simulink model "LCKIE"  (R2020b)
settings: Solver=FixedStepDiscrete  StartTime=0.0  StopTime=Inf  RelTol=1e-3
PostLoadFcn:
  | if any(exist('dsrtsu_mdlpostloadfcn', 'file') ~= 0), dsrtsu_mdlpostloadfcn('Execute', bdroot); end
InitFcn:
  | , if any(exist('rtifpga_mdlclblib', 'file') ~= 0), rtifpga_mdlclblib('Init', bdroot); end,
  | , if any(exist('dsmpb_private', 'file') ~= 0), dsmpb_private('dsmpb_mdlclblib', 'Init', bdroot); end,
PreSaveFcn:
  | , if any(exist('dsmpb_private', 'file') ~= 0), dsmpb_private('dsmpb_mdlclblib', 'PreSave', bdroot); end,
CloseFcn:
  | , if any(exist('dsmpb_private', 'file') ~= 0), dsmpb_private('dsmpb_mdlclblib', 'Close', bdroot); end,
settings Model: DataDictionary=HWA_DDs.sldd  RTICANMMDATA=struct('GeneralSetupData',struct('modelroot','E:\System\ADAS_BaseModel\ADAS_Store\Adas\VSM\LSSState\IE','generalsettings',struct('filesettings',struct('destfolder',struct('Name','RTICANMM_FILES','Check',1),'buildfolder',struct('Name','.','Check',1),'AbsDestfolder',struct('Name','E:\System\ADAS_BaseModel\ADAS_Store\Adas\VSM\LSSState\IE\RTICANMM_FILES'),'AbsBuildfolder',struct('Name','E:\System\ADAS_BaseModel\ADAS_Store\Adas\VSM\LSSState\IE'))),'options',struct('addpaths',1,'rmpaths',1,'addtrcexclusion',false,'cannavigator',struct('checkmonitoring',0),'show_usrtrc',0,'use_usrtrc',0),'advanced',struct('options',ones(1,100)),'MPSetup',{{}},'RTI',struct('Type','DSRT','Ver','4.4','Date','02-Nov-2020'),'modelname','LCKIE','block','LCKIE'))  DSRTSU_INTERNAL_RTIFPGA=170  Creator=GW00164938  LastModifiedBy=GW00164938
settings OptimizationCC: BlockReduction=off  ConditionallyExecuteInputs=off  OptimizeBlockIOStorage=off  BufferReuse=off
settings DebuggingCC: TasksWithSamePriorityMsg=none
settings HardwareCC: ProdBitPerPointer=32  ProdBitPerSizeT=32  ProdBitPerPtrDiffT=32  ProdLargestAtomicInteger=Integer  ProdWordSize=32  ProdHWDeviceType=Custom Processor->Custom
settings ModelReferenceCC: ModelReferenceNumInstancesAllowed=Single
settings SFSimCC: MATLABDynamicMemAlloc=off
settings RTWCC: Description=dSPACE Run-Time Target (for VEOS on Windows and ConfigurationDesk)  SystemTargetFile=dsrt.tlc  GenCodeOnly=on  MakeCommand=make_dsrt  TemplateMakefile=dsrt_default_tmf  RTWVerbose=off
settings CodeAppCC: MaxIdLength=128
settings STFCustomTargetCC: TargetLangStandard=C99 (ISO)  ParMdlRefBuildCompliant=on  ConcurrentExecutionCompliant=off  CPPClassGenCompliant=off  GRTInterface=off  SystemTargetFile=dsrt.tlc
settings GRTTargetCC: CompOptLevelCompliant=off  ConcurrentExecutionCompliant=off  CombineOutputUpdateFcns=off  MatFileLogging=off  CPPClassGenCompliant=off  UseToolchainInfoCompliant=off

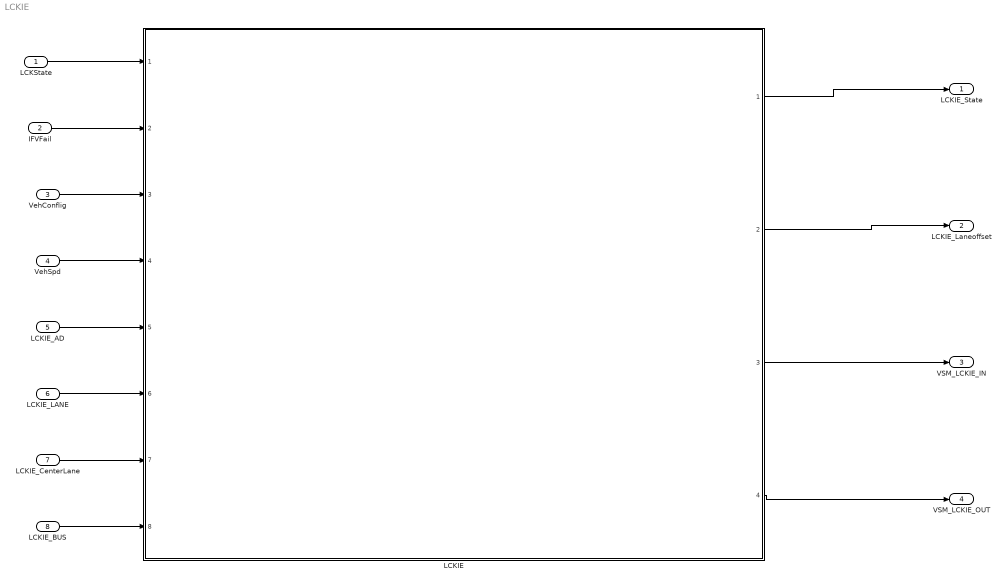
== system LCKIE ==
  LCKState : Inport
  IFVFail : Inport  Port=2
  VehConflig : Inport  Port=3
  VehSpd : Inport  Port=4
  LCKIE_AD : Inport  Port=5  OutDataTypeStr=Bus: LCKIE_AD  BusOutputAsStruct=on
  LCKIE_LANE : Inport  Port=6  OutDataTypeStr=Bus: LCKIE_Lane  BusOutputAsStruct=on
  LCKIE_CenterLane : Inport  Port=7  OutDataTypeStr=Bus: CenterLane  BusOutputAsStruct=on
  LCKIE_BUS : Inport  Port=8  OutDataTypeStr=Bus: TOS_LCKIE_BUS  BusOutputAsStruct=on
  LCKIE : Subsystem  ReferencedSubsystem=PvtSubSys_VSM_LCKIE
  LCKIE_State : Outport
  LCKIE_Laneoffset : Outport  Port=2
  VSM_LCKIE_IN : Outport  Port=3
  VSM_LCKIE_OUT : Outport  Port=4
  wires:
  LCKIE/1 -> LCKIE_State/1
  LCKIE/2 -> LCKIE_Laneoffset/1
  LCKIE/3 -> VSM_LCKIE_IN/1
  LCKIE/4 -> VSM_LCKIE_OUT/1
  VehConflig/1 -> LCKIE/3
  VehSpd/1 -> LCKIE/4
  LCKIE_AD/1 -> LCKIE/5
  LCKIE_CenterLane/1 -> LCKIE/7
  LCKIE_BUS/1 -> LCKIE/8
  IFVFail/1 -> LCKIE/2
  LCKIE_LANE/1 -> LCKIE/6
  LCKState/1 -> LCKIE/1
